simulink model "lab6asim"  (R2022b)
settings: Solver=FixedStepAuto  StartTime=0.0  StopTime=10.0  FixedStep=10/1024  RelTol=1e-3
undefined symbols (not defined in the file or in its folder): lutdata, lutix
settings Model: Creator=andjog  LastModifiedBy=andjog

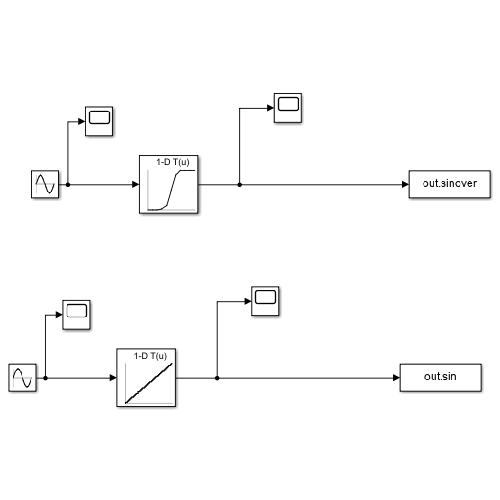
[thumbnail: Simulink's stored preview of the top-level diagram]
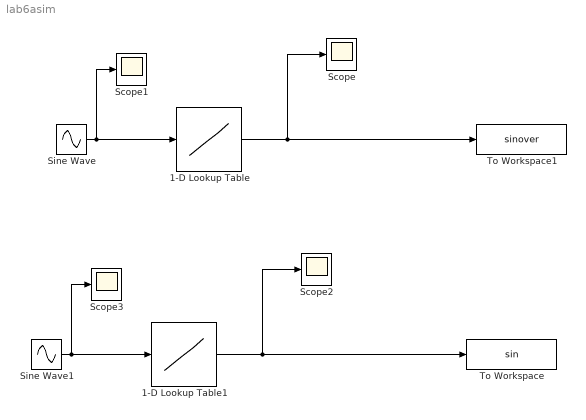
== system lab6asim ==
  1-D Lookup Table : Lookup_n-D  NumberOfTableDimensions=1  BreakpointsForDimension1=lutix(2^7*2^5)  Table=lutdata(2^7*2^5)  InternalRulePriority=Speed  RndMeth=Simplest
  1-D Lookup Table1 : Lookup_n-D  NumberOfTableDimensions=1  BreakpointsForDimension1=lutix(2^7)  Table=lutdata(2^7)  InternalRulePriority=Speed  RndMeth=Simplest
  Scope{,1..3} (4 alike) : Scope
  Sine Wave : Sin  Frequency=pi  SampleTime=0
  Sine Wave1 : Sin  Frequency=pi  SampleTime=0
  To Workspace : ToWorkspace  VariableName=sin  SaveFormat=Structure With Time  SampleTime=-1
  To Workspace1 : ToWorkspace  VariableName=sinover  SaveFormat=Structure With Time  SampleTime=-1
  wires:
  Sine Wave/1 -> 1-D Lookup Table/1, Scope1/1
  1-D Lookup Table/1 -> To Workspace1/1, Scope/1
  1-D Lookup Table1/1 -> To Workspace/1, Scope2/1
  Sine Wave1/1 -> 1-D Lookup Table1/1, Scope3/1
